simulink model "abEPMAFPLL"  (R2020b)
settings: Solver=FixedStepAuto  StartTime=0.0  StopTime=5  FixedStep=Ts  MaxStep=1e-5  RelTol=1e-3
values from neighbouring files (symbols this model uses):
  N = T_MAF/Ts    (= 200)    [maf_filter.m]
undefined symbols (not defined in the file or in its folder): A_frq_step, A_phase_step, f_rad, k_phi, ki, kp, t_frq_step, t_phase_step, V_g, var_noise
libraries: simulink x7, bach_library x3
settings Model: Creator=Martin  LastModifiedBy=Kasper Laustsen

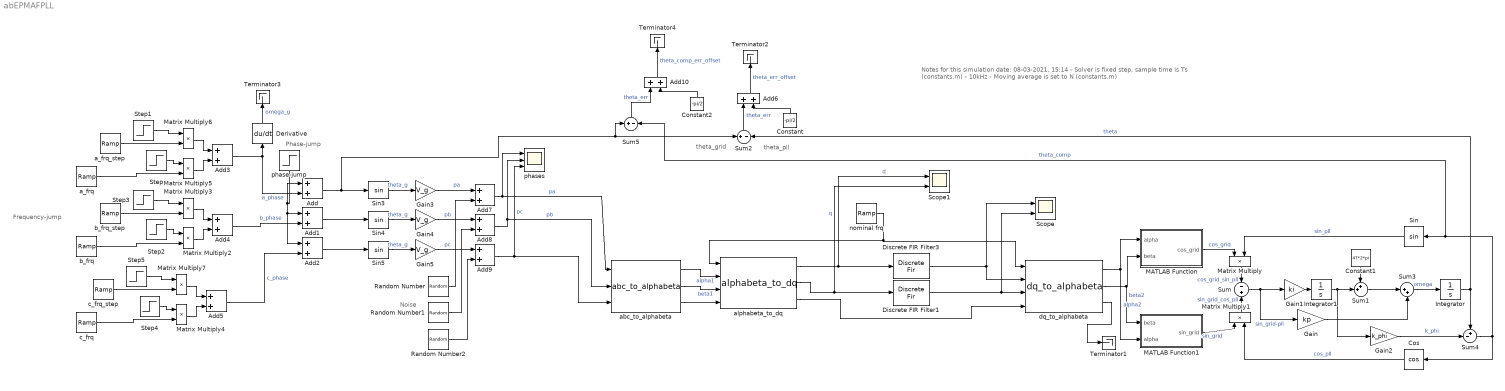
== system abEPMAFPLL ==
  note: Notes for this simulation
      |
      | date: 08-03-2021, 15:14
      | - Solver is fixed step, sample time is Ts (constants.m) - 10kHz
      | - Moving average is set to N (constants.m)
  note: Noise
  note: Phase-jump
  note: theta_grid
  note: theta_pll
  note: Frequency-jump
  Add{,1..10} (11 alike) : Sum
  Constant : Constant  Value=-pi/2
  Constant1 : Constant  Value=47*2*pi
  Constant2 : Constant  Value=-pi/2
  Cos : Trigonometry  Operator=cos
  Derivative : Derivative
  Discrete FIR Filter1 : DiscreteFir  Coefficients=[ones(1,N).*1/N]
  Discrete FIR Filter3 : DiscreteFir  Coefficients=[ones(1,N).*1/N]
  Gain : Gain  Gain=kp
  Gain1 : Gain  Gain=ki
  Gain2 : Gain  Gain=k_phi
  Gain3 : Gain  Gain=V_g
  Gain4 : Gain  Gain=V_g
  Gain5 : Gain  Gain=V_g
  Integrator : Integrator
  Integrator1 : Integrator
  MATLAB Function : MATLAB Function  TreatAsAtomicUnit=on
  MATLAB Function1 : MATLAB Function  TreatAsAtomicUnit=on
  Matrix Multiply{,1..7} (8 alike) : Product
  Random Number : RandomNumber  Variance=var_noise
  Random Number1 : RandomNumber  Variance=var_noise  Seed=1
  Random Number2 : RandomNumber  Variance=var_noise  Seed=2
  Scope : Scope  NumInputPorts=2
  Scope1 : Scope  NumInputPorts=2
  Sin{,3..5} (4 alike) : Trigonometry
  Step : Step  Time=t_frq_step  Before=1  After=0  SampleTime=0
  Step1 : Step  Time=t_frq_step  SampleTime=0
  Step2 : Step  Time=t_frq_step  Before=1  After=0  SampleTime=0
  Step3 : Step  Time=t_frq_step  SampleTime=0
  Step4 : Step  Time=t_frq_step  Before=1  After=0  SampleTime=0
  Step5 : Step  Time=t_frq_step  SampleTime=0
  Sum : Sum  Inputs=-|+
  Sum1 : Sum  Inputs=++|
  Sum2 : Sum  Inputs=+|-
  Sum3 : Sum  Inputs=|++
  Sum4 : Sum  Inputs=+-|
  Sum5 : Sum  Inputs=+|-
  Terminator{1..4} (4 alike) : Terminator
  a_frq : simulink/Sources/Ramp  slope=f_rad  start=0  InitialOutput=0
  a_frq_step : simulink/Sources/Ramp  slope=f_rad*A_frq_step  start=t_frq_step  InitialOutput=t_frq_step*f_rad
  abc_to_alphabeta : bach_library/abc_to_alphabeta  SystemSampleTime=-1  VariantActivationTime=update diagram  Latency=0  AutoFrameSizeCalculation=off
  alphabeta_to_dq : bach_library/alphabeta_to_dq  SystemSampleTime=-1  VariantActivationTime=update diagram  Latency=0  AutoFrameSizeCalculation=off
  b_frq : simulink/Sources/Ramp  slope=f_rad  start=0  InitialOutput=f_rad/3
  b_frq_step : simulink/Sources/Ramp  slope=f_rad*A_frq_step  start=t_frq_step  InitialOutput=t_frq_step*f_rad+f_rad/3
  c_frq : simulink/Sources/Ramp  slope=f_rad  start=0  InitialOutput=f_rad*2/3
  c_frq_step : simulink/Sources/Ramp  slope=f_rad*A_frq_step  start=t_frq_step  InitialOutput=t_frq_step*f_rad+f_rad*2/3
  dq_to_alphabeta : bach_library/dq_to_alphabeta  SystemSampleTime=-1  VariantActivationTime=update diagram  Latency=0  AutoFrameSizeCalculation=off
  nominal frq : simulink/Sources/Ramp  slope=47*2*pi  start=0  InitialOutput=0
  phase-jump : Step  Time=t_phase_step  After=A_phase_step  SampleTime=0
  phases : Scope  NumInputPorts=3
  wires:
  Derivative/1 -> Terminator3/1  "omega_g"
  Step2/1 -> Matrix Multiply2/1
  MATLAB Function/1(cos_grid) -> Matrix Multiply/1  "cos_grid"
  Constant/1 -> Add6/2
  Step/1 -> Matrix Multiply5/1
  Sin5/1 -> Gain5/1  "theta_g"
  Sin3/1 -> Gain3/1  "theta_g"
  Step1/1 -> Matrix Multiply6/1
  a_frq/1 -> Matrix Multiply5/2
  Step4/1 -> Matrix Multiply4/1
  Matrix Multiply2/1 -> Add4/2
  Matrix Multiply7/1 -> Add5/1
  Matrix Multiply6/1 -> Add3/1
  a_frq_step/1 -> Matrix Multiply6/2
  Add6/1 -> Terminator2/1  "theta_err_offset"
  Sum2/1 -> Add6/1  "theta_err"
  Sin/1 -> Matrix Multiply/2  "sin_pll"
  Sum/1 -> Gain1/1, Gain/1  "sin_grid-pll"
  Add1/1 -> Sin4/1
  phase-jump/1 -> Add/1, Add2/1, Add1/1
  Matrix Multiply4/1 -> Add5/2
  Add4/1 -> Add1/2  "b_phase"
  Add9/1 -> abc_to_alphabeta/3, phases/3  "pc"
  Add5/1 -> Add2/2  "c_phase"
  Cos/1 -> Matrix Multiply1/2  "cos_pll"
  Add7/1 -> abc_to_alphabeta/1, phases/1  "pa"
  Matrix Multiply/1 -> Sum/1  "cos_grid_sin_pll"
  Add8/1 -> phases/2, abc_to_alphabeta/2  "pb"
  Add/1 -> Sum5/1, Sum2/1, Sin3/1
  Random Number/1 -> Add7/2
  Step3/1 -> Matrix Multiply3/1
  Add2/1 -> Sin5/1
  Gain3/1 -> Add7/1  "pa"
  c_frq/1 -> Matrix Multiply4/2
  Matrix Multiply5/1 -> Add3/2
  Add3/1 -> Add/2, Derivative/1  "a_phase"
  Matrix Multiply3/1 -> Add4/1
  Sin4/1 -> Gain4/1  "theta_g"
  MATLAB Function1/1(sin_grid) -> Matrix Multiply1/1  "sin_grid"
  Matrix Multiply1/1 -> Sum/2  "sin_grid_cos_pll"
  Random Number1/1 -> Add8/2
  b_frq_step/1 -> Matrix Multiply3/2
  Random Number2/1 -> Add9/2
  b_frq/1 -> Matrix Multiply2/2
  c_frq_step/1 -> Matrix Multiply7/2
  Gain5/1 -> Add9/1  "pc"
  Gain4/1 -> Add8/1  "pb"
  Step5/1 -> Matrix Multiply7/1
  Gain1/1 -> Integrator1/1
  Gain/1 -> Sum3/2
  Integrator1/1 -> Sum1/2, Gain2/1
  Integrator/1 -> Sum2/2, Sum4/1  "theta"
  Gain2/1 -> Sum4/2  "k_phi"
  Sum4/1 -> Cos/1, Sum5/2, Sin/1  "theta_comp"
  abc_to_alphabeta/3 -> alphabeta_to_dq/4
  dq_to_alphabeta/1 -> MATLAB Function/1(alpha), MATLAB Function1/2(alpha)  "alpha2"
  dq_to_alphabeta/2 -> MATLAB Function1/1(beta), MATLAB Function/2(beta)  "beta2"
  nominal frq/1 -> dq_to_alphabeta/1, alphabeta_to_dq/1
  abc_to_alphabeta/1 -> alphabeta_to_dq/2  "alpha1"
  abc_to_alphabeta/2 -> alphabeta_to_dq/3  "beta1"
  alphabeta_to_dq/2 -> Discrete FIR Filter1/1, Scope1/2  "q"
  alphabeta_to_dq/1 -> Scope1/1, Discrete FIR Filter3/1  "d"
  Discrete FIR Filter3/1 -> Scope/1, dq_to_alphabeta/2
  Discrete FIR Filter1/1 -> Scope/2, dq_to_alphabeta/3
  alphabeta_to_dq/3 -> dq_to_alphabeta/4
  Sum1/1 -> Sum3/1
  Constant1/1 -> Sum1/1
  Sum3/1 -> Integrator/1  "omega"
  dq_to_alphabeta/3 -> Terminator1/1
  Add10/1 -> Terminator4/1  "theta_comp_err_offset"
  Sum5/1 -> Add10/1  "theta_err"
  Constant2/1 -> Add10/2

== matlab function abEPMAFPLL/MATLAB Function ==
  data: alpha input; cos_grid output; beta input
function cos_grid = cos_grid(alpha, beta)

cos_grid = alpha/sqrt(alpha^2+beta^2);

== matlab function abEPMAFPLL/MATLAB Function1 ==
  data: beta input; alpha input; sin_grid output
function sin_grid = sin_grid(beta, alpha)

sin_grid = beta/sqrt(alpha^2+beta^2);
